simulink model "Brown_6DOF_Sim_Wrapper_EUL"  (R2025b)
settings: Solver=VariableStepAuto  StartTime=0.0  StopTime=10  RelTol=1e-3
values from neighbouring files (symbols this model uses):
  controller_airspeed_cmd_base = norm(V_init)    [Brown_6DOF_Init_main.m]    (also in Full_Sim_Init.m; Init_Main.m)
  controller_airspeed_step = 0.0    (= 0)    [Brown_6DOF_Init_main.m]    (also in Full_Sim_Init.m; Init_Main.m)
  controller_bank_cmd_base = eul_init(1)    [Brown_6DOF_Init_main.m]    (also in Full_Sim_Init.m; Init_Main.m)
  controller_bank_step = 0.0    (= 0)    [Brown_6DOF_Init_main.m]    (also in Full_Sim_Init.m; Init_Main.m)
  controller_enable = false    [Brown_6DOF_Init_main.m]    (also in Full_Sim_Init.m; Init_Main.m; Run_Main.m)
  controller_integrator_limit = 200.0    (= 200)    [Brown_6DOF_Init_main.m]    (also in Full_Sim_Init.m; Init_Main.m)
  controller_k_p_damp = 0.0    (= 0)    [Brown_6DOF_Init_main.m]    (also in Full_Sim_Init.m; Init_Main.m)
  controller_k_phi_i = 0.0    (= 0)    [Brown_6DOF_Init_main.m]    (also in Full_Sim_Init.m; Init_Main.m)
  controller_k_phi_p = 0.0    (= 0)    [Brown_6DOF_Init_main.m]    (also in Full_Sim_Init.m; Init_Main.m)
  controller_k_q_damp = 0.0    (= 0)    [Brown_6DOF_Init_main.m]    (also in Full_Sim_Init.m; Init_Main.m)
  controller_k_r_damp = 0.0    (= 0)    [Brown_6DOF_Init_main.m]    (also in Full_Sim_Init.m; Init_Main.m)
  controller_k_v_i = 0.0    (= 0)    [Brown_6DOF_Init_main.m]    (also in Full_Sim_Init.m; Init_Main.m)
  controller_k_v_p = 0.0    (= 0)    [Brown_6DOF_Init_main.m]    (also in Full_Sim_Init.m; Init_Main.m)
  controller_mode = 0    [Brown_6DOF_Init_main.m]    (also in Full_Sim_Init.m; Init_Main.m = 1; Run_Main.m = 1)
  controller_rpm_delta_limit = 2000.0    (= 2000)    [Brown_6DOF_Init_main.m]    (also in Full_Sim_Init.m; Init_Main.m)
  controller_sample_time = 0.01    [Brown_6DOF_Init_main.m]    (also in Full_Sim_Init.m; HW356_simple_demos_live_source.m; Init_Main.m)
  controller_step_time = 1.0    (= 1)    [Brown_6DOF_Init_main.m]    (also in Full_Sim_Init.m; Init_Main.m)
  controller_surface_limit_rad = deg2rad(25.0)    [Brown_6DOF_Init_main.m]    (also in Full_Sim_Init.m; Init_Main.m)
  controller_trim_delta_a = 0.0    (= 0)    [Brown_6DOF_Init_main.m]    (also in Full_Sim_Init.m; Init_Main.m)
  controller_trim_delta_e = 0.0    (= 0)    [Brown_6DOF_Init_main.m]    (also in Full_Sim_Init.m; Init_Main.m)
  controller_trim_delta_f = 0.0    (= 0)    [Brown_6DOF_Init_main.m]    (also in Full_Sim_Init.m; Init_Main.m)
  controller_trim_delta_r = 0.0    (= 0)    [Brown_6DOF_Init_main.m]    (also in Full_Sim_Init.m; Init_Main.m)
  controller_trim_motor_rpm_cmd = Motor_RPMs(:)    [Brown_6DOF_Init_main.m]    (also in Full_Sim_Init.m = zeros(12, 1); Init_Main.m = zeros(4, 1))
  controller_trim_tilt_angles_cmd = Tilt_angles(:)    [Brown_6DOF_Init_main.m]    (also in Full_Sim_Init.m = front_tilt_group * ones(6, 1); Init_Main.m = front_tilt_group * ones(numel(Tilt_angles), 1))
  estimator_enable = true    [Brown_6DOF_Init_main.m]    (also in Full_Sim_Init.m)
  estimator_init_eul = eul_init    [Brown_6DOF_Init_main.m]    (also in Full_Sim_Init.m)
  estimator_k_acc = 3.0    (= 3)    [Brown_6DOF_Init_main.m]    (also in Full_Sim_Init.m)
  estimator_k_att = 0.0    (= 0)    [Brown_6DOF_Init_main.m]    (also in Full_Sim_Init.m)
  estimator_k_mag = 1.5    [Brown_6DOF_Init_main.m]    (also in Full_Sim_Init.m)
  estimator_sample_time = controller_sample_time    (= 0.01)    [Brown_6DOF_Init_main.m]    (also in Full_Sim_Init.m)
  mag_ned = [0.23; 0.00; 0.43]    [Brown_6DOF_Init_main.m]    (also in Full_Sim_Init.m)
  sensor_accel_bias = zeros(3, 1)    [Brown_6DOF_Init_main.m]    (also in Full_Sim_Init.m; Init_Main.m = [0; 0; 0])
  sensor_accel_sigma = [0.05; 0.05; 0.05]    [Brown_6DOF_Init_main.m]    (also in Full_Sim_Init.m; Init_Main.m = [0; 0; 0])
  sensor_airdata_bias = zeros(3, 1)    [Brown_6DOF_Init_main.m]    (also in Full_Sim_Init.m; Init_Main.m = [0; 0; 0])
  sensor_airdata_sigma = [0.20; deg2rad(0.10); deg2rad(0.10)]    [Brown_6DOF_Init_main.m]    (also in Full_Sim_Init.m; Init_Main.m = [0; 0; 0])
  sensor_attitude_bias = zeros(3, 1)    [Brown_6DOF_Init_main.m]    (also in Full_Sim_Init.m)
  sensor_attitude_sigma = deg2rad([0.10; 0.10; 0.15])    [Brown_6DOF_Init_main.m]    (also in Full_Sim_Init.m)
  sensor_enable_bias = true    [Brown_6DOF_Init_main.m]    (also in Full_Sim_Init.m)
  sensor_enable_noise = true    [Brown_6DOF_Init_main.m]    (also in Full_Sim_Init.m)
  sensor_gps_pos_bias = zeros(3, 1)    [Brown_6DOF_Init_main.m]    (also in Full_Sim_Init.m)
  sensor_gps_pos_sigma = [0.50; 0.50; 0.50]    [Brown_6DOF_Init_main.m]    (also in Full_Sim_Init.m)
  sensor_gps_vel_bias = zeros(3, 1)    [Brown_6DOF_Init_main.m]    (also in Full_Sim_Init.m)
  sensor_gps_vel_sigma = [0.05; 0.05; 0.05]    [Brown_6DOF_Init_main.m]    (also in Full_Sim_Init.m)
  sensor_gyro_bias = zeros(3, 1)    [Brown_6DOF_Init_main.m]    (also in Full_Sim_Init.m; Init_Main.m = [0; 0; 0])
  sensor_gyro_sigma = deg2rad([0.05; 0.05; 0.05])    [Brown_6DOF_Init_main.m]    (also in Full_Sim_Init.m; Init_Main.m = [0; 0; 0])
  sensor_mag_bias = zeros(3, 1)    [Brown_6DOF_Init_main.m]    (also in Full_Sim_Init.m; Init_Main.m = [0; 0; 0])
  sensor_mag_sigma = [0.005; 0.005; 0.005]    [Brown_6DOF_Init_main.m]    (also in Full_Sim_Init.m; Init_Main.m = [0; 0; 0])
  sensor_sample_time = controller_sample_time    (= 0.01)    [Brown_6DOF_Init_main.m]    (also in Full_Sim_Init.m; Init_Main.m)
undefined symbols (not defined in the file or in its folder): trim_front_collective_rpm, trim_rear_collective_rpm
settings Model: Creator=zbrown  LastModifiedBy=zbrown

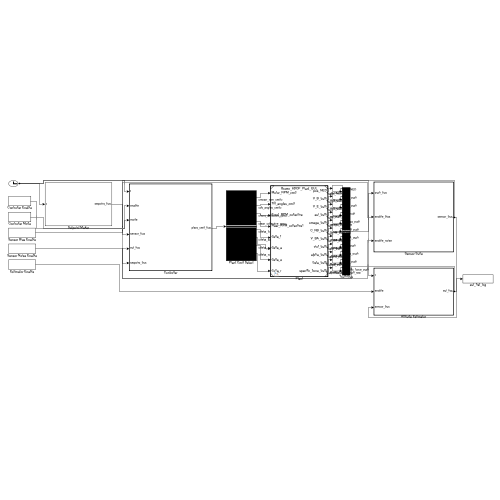
[thumbnail: Simulink's stored preview of the top-level diagram]
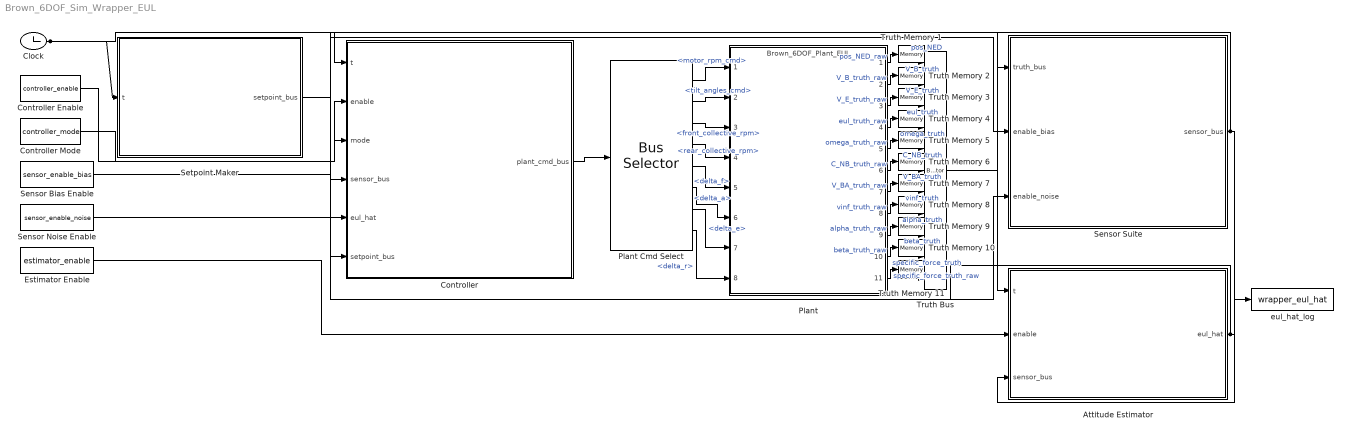
== system Brown_6DOF_Sim_Wrapper_EUL ==
  Attitude Estimator : Subsystem  TreatAsAtomicUnit=on  SystemSampleTime=estimator_sample_time
  Clock : Clock
  Controller : Subsystem  TreatAsAtomicUnit=on  SystemSampleTime=controller_sample_time
  Controller Enable : Constant  Value=controller_enable
  Controller Mode : Constant  Value=controller_mode
  Estimator Enable : Constant  Value=estimator_enable
  Plant : ModelReference  ModelNameDialog=Brown_6DOF_Plant_EUL  SimulationMode=Normal  ModelReferenceVersion=1.34
  Plant Cmd Select : BusSelector  OutputSignals=motor_rpm_cmd,tilt_angles_cmd,front_collective_rpm,rear_collective_rpm,delta_f,delta_a,delta_e,delta_r
  Sensor Bias Enable : Constant  Value=sensor_enable_bias
  Sensor Noise Enable : Constant  Value=sensor_enable_noise
  Sensor Suite : Subsystem  TreatAsAtomicUnit=on  SystemSampleTime=sensor_sample_time
  Setpoint Maker : Subsystem
  Truth Bus : BusCreator  Inputs=11
  Truth Memory {1..11} (11 alike) : Memory
  eul_hat_log : ToWorkspace  VariableName=wrapper_eul_hat  SampleTime=-1
  wires:
  Clock/1 -> Setpoint Maker/1(t), Controller/1(t), Attitude Estimator/1(t)
  Controller Enable/1 -> Controller/2(enable)
  Controller Mode/1 -> Controller/3(mode)
  Setpoint Maker/1(setpoint_bus) -> Controller/6(setpoint_bus)
  Controller/1(plant_cmd_bus) -> Plant Cmd Select/1
  Plant Cmd Select/1 -> Plant/1  "<motor_rpm_cmd>"
  Plant Cmd Select/2 -> Plant/2  "<tilt_angles_cmd>"
  Plant Cmd Select/3 -> Plant/3  "<front_collective_rpm>"
  Plant Cmd Select/4 -> Plant/4  "<rear_collective_rpm>"
  Plant Cmd Select/5 -> Plant/5  "<delta_f>"
  Plant Cmd Select/6 -> Plant/6  "<delta_a>"
  Plant Cmd Select/7 -> Plant/7  "<delta_e>"
  Plant Cmd Select/8 -> Plant/8  "<delta_r>"
  Plant/1 -> Truth Memory 1/1  "pos_NED_raw"
  Truth Memory 1/1 -> Truth Bus/1  "pos_NED"
  Plant/2 -> Truth Memory 2/1  "V_B_truth_raw"
  Truth Memory 2/1 -> Truth Bus/2  "V_B_truth"
  Plant/3 -> Truth Memory 3/1  "V_E_truth_raw"
  Truth Memory 3/1 -> Truth Bus/3  "V_E_truth"
  Plant/4 -> Truth Memory 4/1  "eul_truth_raw"
  Truth Memory 4/1 -> Truth Bus/4  "eul_truth"
  Plant/5 -> Truth Memory 5/1  "omega_truth_raw"
  Truth Memory 5/1 -> Truth Bus/5  "omega_truth"
  Plant/6 -> Truth Memory 6/1  "C_NB_truth_raw"
  Truth Memory 6/1 -> Truth Bus/6  "C_NB_truth"
  Plant/7 -> Truth Memory 7/1  "V_BA_truth_raw"
  Truth Memory 7/1 -> Truth Bus/7  "V_BA_truth"
  Plant/8 -> Truth Memory 8/1  "vinf_truth_raw"
  Truth Memory 8/1 -> Truth Bus/8  "vinf_truth"
  Plant/9 -> Truth Memory 9/1  "alpha_truth_raw"
  Truth Memory 9/1 -> Truth Bus/9  "alpha_truth"
  Plant/10 -> Truth Memory 10/1  "beta_truth_raw"
  Truth Memory 10/1 -> Truth Bus/10  "beta_truth"
  Plant/11 -> Truth Memory 11/1  "specific_force_truth_raw"
  Truth Memory 11/1 -> Truth Bus/11  "specific_force_truth"
  Truth Bus/1 -> Sensor Suite/1(truth_bus)
  Sensor Bias Enable/1 -> Sensor Suite/2(enable_bias)
  Sensor Noise Enable/1 -> Sensor Suite/3(enable_noise)
  Sensor Suite/1(sensor_bus) -> Attitude Estimator/3(sensor_bus), Controller/4(sensor_bus)
  Estimator Enable/1 -> Attitude Estimator/2(enable)
  Attitude Estimator/1(eul_hat) -> Controller/5(eul_hat), eul_hat_log/1

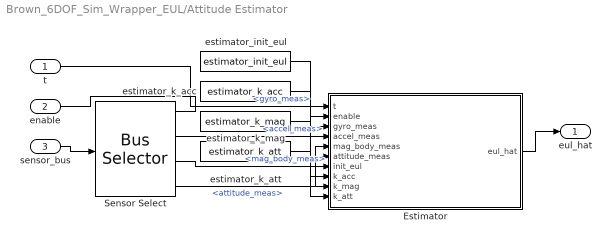
== system Brown_6DOF_Sim_Wrapper_EUL/Attitude Estimator ==
  t : Inport
  enable : Inport  Port=2
  sensor_bus : Inport  Port=3
  Estimator : MATLAB Function  TreatAsAtomicUnit=on
  Sensor Select : BusSelector  OutputSignals=gyro_meas,accel_meas,mag_body_meas,attitude_meas
  estimator_init_eul : Constant  Value=estimator_init_eul
  estimator_k_acc : Constant  Value=estimator_k_acc
  estimator_k_att : Constant  Value=estimator_k_att
  estimator_k_mag : Constant  Value=estimator_k_mag
  eul_hat : Outport
  wires:
  ? -> ?
  t/1 -> Estimator/1(t)
  enable/1 -> Estimator/2(enable)
  sensor_bus/1 -> Sensor Select/1
  Sensor Select/1 -> Estimator/3(gyro_meas)  "<gyro_meas>"
  Sensor Select/2 -> Estimator/4(accel_meas)  "<accel_meas>"
  Sensor Select/3 -> Estimator/5(mag_body_meas)  "<mag_body_meas>"
  Sensor Select/4 -> Estimator/6(attitude_meas)  "<attitude_meas>"
  estimator_init_eul/1 -> Estimator/7(init_eul)
  estimator_k_acc/1 -> Estimator/8(k_acc)
  estimator_k_mag/1 -> Estimator/9(k_mag)
  estimator_k_att/1 -> Estimator/10(k_att)
  Estimator/1(eul_hat) -> eul_hat/1

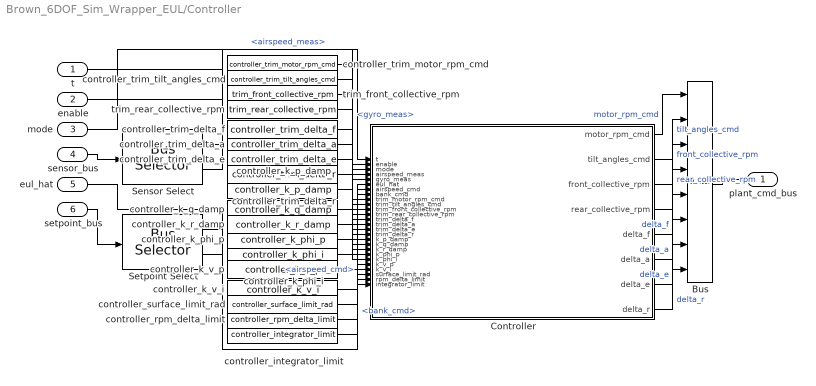
== system Brown_6DOF_Sim_Wrapper_EUL/Controller ==
  t : Inport
  enable : Inport  Port=2
  mode : Inport  Port=3
  sensor_bus : Inport  Port=4
  eul_hat : Inport  Port=5
  setpoint_bus : Inport  Port=6
  Bus : BusCreator  Inputs=8
  Controller : MATLAB Function  TreatAsAtomicUnit=on
  Sensor Select : BusSelector  OutputSignals=airspeed_meas,gyro_meas
  Setpoint Select : BusSelector  OutputSignals=airspeed_cmd,bank_cmd
  controller_integrator_limit : Constant  Value=controller_integrator_limit
  controller_k_p_damp : Constant  Value=controller_k_p_damp
  controller_k_phi_i : Constant  Value=controller_k_phi_i
  controller_k_phi_p : Constant  Value=controller_k_phi_p
  controller_k_q_damp : Constant  Value=controller_k_q_damp
  controller_k_r_damp : Constant  Value=controller_k_r_damp
  controller_k_v_i : Constant  Value=controller_k_v_i
  controller_k_v_p : Constant  Value=controller_k_v_p
  controller_rpm_delta_limit : Constant  Value=controller_rpm_delta_limit
  controller_surface_limit_rad : Constant  Value=controller_surface_limit_rad
  controller_trim_delta_a : Constant  Value=controller_trim_delta_a
  controller_trim_delta_e : Constant  Value=controller_trim_delta_e
  controller_trim_delta_f : Constant  Value=controller_trim_delta_f
  controller_trim_delta_r : Constant  Value=controller_trim_delta_r
  controller_trim_motor_rpm_cmd : Constant  Value=controller_trim_motor_rpm_cmd
  controller_trim_tilt_angles_cmd : Constant  Value=controller_trim_tilt_angles_cmd
  trim_front_collective_rpm : Constant  Value=trim_front_collective_rpm
  trim_rear_collective_rpm : Constant  Value=trim_rear_collective_rpm
  plant_cmd_bus : Outport
  wires:
  ? -> ?
  t/1 -> Controller/1(t)
  enable/1 -> Controller/2(enable)
  mode/1 -> Controller/3(mode)
  sensor_bus/1 -> Sensor Select/1
  setpoint_bus/1 -> Setpoint Select/1
  eul_hat/1 -> Controller/6(eul_hat)
  Sensor Select/1 -> Controller/4(airspeed_meas)  "<airspeed_meas>"
  Sensor Select/2 -> Controller/5(gyro_meas)  "<gyro_meas>"
  Setpoint Select/1 -> Controller/7(airspeed_cmd)  "<airspeed_cmd>"
  Setpoint Select/2 -> Controller/8(bank_cmd)  "<bank_cmd>"
  controller_trim_motor_rpm_cmd/1 -> Controller/9(trim_motor_rpm_cmd)
  controller_trim_tilt_angles_cmd/1 -> Controller/10(trim_tilt_angles_cmd)
  trim_front_collective_rpm/1 -> Controller/11(trim_front_collective_rpm)
  trim_rear_collective_rpm/1 -> Controller/12(trim_rear_collective_rpm)
  controller_trim_delta_f/1 -> Controller/13(trim_delta_f)
  controller_trim_delta_a/1 -> Controller/14(trim_delta_a)
  controller_trim_delta_e/1 -> Controller/15(trim_delta_e)
  controller_trim_delta_r/1 -> Controller/16(trim_delta_r)
  controller_k_p_damp/1 -> Controller/17(k_p_damp)
  controller_k_q_damp/1 -> Controller/18(k_q_damp)
  controller_k_r_damp/1 -> Controller/19(k_r_damp)
  controller_k_phi_p/1 -> Controller/20(k_phi_p)
  controller_k_phi_i/1 -> Controller/21(k_phi_i)
  controller_k_v_p/1 -> Controller/22(k_v_p)
  controller_k_v_i/1 -> Controller/23(k_v_i)
  controller_surface_limit_rad/1 -> Controller/24(surface_limit_rad)
  controller_rpm_delta_limit/1 -> Controller/25(rpm_delta_limit)
  controller_integrator_limit/1 -> Controller/26(integrator_limit)
  Controller/1(motor_rpm_cmd) -> Bus/1  "motor_rpm_cmd"
  Controller/2(tilt_angles_cmd) -> Bus/2  "tilt_angles_cmd"
  Controller/3(front_collective_rpm) -> Bus/3  "front_collective_rpm"
  Controller/4(rear_collective_rpm) -> Bus/4  "rear_collective_rpm"
  Controller/5(delta_f) -> Bus/5  "delta_f"
  Controller/6(delta_a) -> Bus/6  "delta_a"
  Controller/7(delta_e) -> Bus/7  "delta_e"
  Controller/8(delta_r) -> Bus/8  "delta_r"
  Bus/1 -> plant_cmd_bus/1

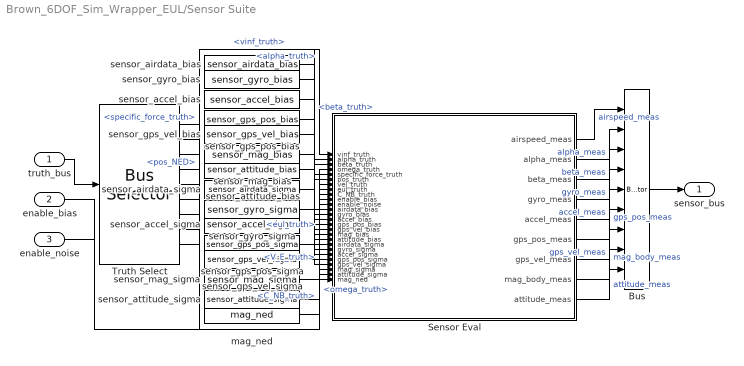
== system Brown_6DOF_Sim_Wrapper_EUL/Sensor Suite ==
  truth_bus : Inport
  enable_bias : Inport  Port=2
  enable_noise : Inport  Port=3
  Bus : BusCreator  Inputs=9
  Sensor Eval : MATLAB Function  TreatAsAtomicUnit=on
  Truth Select : BusSelector  OutputSignals=vinf_truth,alpha_truth,beta_truth,omega_truth,specific_force_truth,pos_NED,V_E_truth,eul_truth,C_NB_truth
  mag_ned : Constant  Value=mag_ned
  sensor_accel_bias : Constant  Value=sensor_accel_bias
  sensor_accel_sigma : Constant  Value=sensor_accel_sigma
  sensor_airdata_bias : Constant  Value=sensor_airdata_bias
  sensor_airdata_sigma : Constant  Value=sensor_airdata_sigma
  sensor_attitude_bias : Constant  Value=sensor_attitude_bias
  sensor_attitude_sigma : Constant  Value=sensor_attitude_sigma
  sensor_gps_pos_bias : Constant  Value=sensor_gps_pos_bias
  sensor_gps_pos_sigma : Constant  Value=sensor_gps_pos_sigma
  sensor_gps_vel_bias : Constant  Value=sensor_gps_vel_bias
  sensor_gps_vel_sigma : Constant  Value=sensor_gps_vel_sigma
  sensor_gyro_bias : Constant  Value=sensor_gyro_bias
  sensor_gyro_sigma : Constant  Value=sensor_gyro_sigma
  sensor_mag_bias : Constant  Value=sensor_mag_bias
  sensor_mag_sigma : Constant  Value=sensor_mag_sigma
  sensor_bus : Outport
  wires:
  ? -> ?
  truth_bus/1 -> Truth Select/1
  Truth Select/1 -> Sensor Eval/1(vinf_truth)  "<vinf_truth>"
  Truth Select/2 -> Sensor Eval/2(alpha_truth)  "<alpha_truth>"
  Truth Select/3 -> Sensor Eval/3(beta_truth)  "<beta_truth>"
  Truth Select/4 -> Sensor Eval/4(omega_truth)  "<omega_truth>"
  Truth Select/5 -> Sensor Eval/5(specific_force_truth)  "<specific_force_truth>"
  Truth Select/6 -> Sensor Eval/6(pos_truth)  "<pos_NED>"
  Truth Select/7 -> Sensor Eval/7(vel_truth)  "<V_E_truth>"
  Truth Select/8 -> Sensor Eval/8(eul_truth)  "<eul_truth>"
  Truth Select/9 -> Sensor Eval/9(C_NB_truth)  "<C_NB_truth>"
  enable_bias/1 -> Sensor Eval/10(enable_bias)
  enable_noise/1 -> Sensor Eval/11(enable_noise)
  sensor_airdata_bias/1 -> Sensor Eval/12(airdata_bias)
  sensor_gyro_bias/1 -> Sensor Eval/13(gyro_bias)
  sensor_accel_bias/1 -> Sensor Eval/14(accel_bias)
  sensor_gps_pos_bias/1 -> Sensor Eval/15(gps_pos_bias)
  sensor_gps_vel_bias/1 -> Sensor Eval/16(gps_vel_bias)
  sensor_mag_bias/1 -> Sensor Eval/17(mag_bias)
  sensor_attitude_bias/1 -> Sensor Eval/18(attitude_bias)
  sensor_airdata_sigma/1 -> Sensor Eval/19(airdata_sigma)
  sensor_gyro_sigma/1 -> Sensor Eval/20(gyro_sigma)
  sensor_accel_sigma/1 -> Sensor Eval/21(accel_sigma)
  sensor_gps_pos_sigma/1 -> Sensor Eval/22(gps_pos_sigma)
  sensor_gps_vel_sigma/1 -> Sensor Eval/23(gps_vel_sigma)
  sensor_mag_sigma/1 -> Sensor Eval/24(mag_sigma)
  sensor_attitude_sigma/1 -> Sensor Eval/25(attitude_sigma)
  mag_ned/1 -> Sensor Eval/26(mag_ned)
  Sensor Eval/1(airspeed_meas) -> Bus/1  "airspeed_meas"
  Sensor Eval/2(alpha_meas) -> Bus/2  "alpha_meas"
  Sensor Eval/3(beta_meas) -> Bus/3  "beta_meas"
  Sensor Eval/4(gyro_meas) -> Bus/4  "gyro_meas"
  Sensor Eval/5(accel_meas) -> Bus/5  "accel_meas"
  Sensor Eval/6(gps_pos_meas) -> Bus/6  "gps_pos_meas"
  Sensor Eval/7(gps_vel_meas) -> Bus/7  "gps_vel_meas"
  Sensor Eval/8(mag_body_meas) -> Bus/8  "mag_body_meas"
  Sensor Eval/9(attitude_meas) -> Bus/9  "attitude_meas"
  Bus/1 -> sensor_bus/1

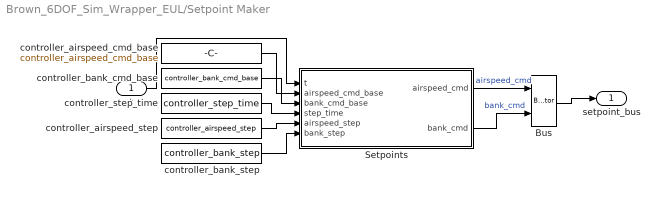
== system Brown_6DOF_Sim_Wrapper_EUL/Setpoint Maker ==
  t : Inport
  Bus : BusCreator  Inputs=2
  Setpoints : MATLAB Function  TreatAsAtomicUnit=on
  controller_airspeed_cmd_base : Constant  Value=controller_airspeed_cmd_base
  controller_airspeed_step : Constant  Value=controller_airspeed_step
  controller_bank_cmd_base : Constant  Value=controller_bank_cmd_base
  controller_bank_step : Constant  Value=controller_bank_step
  controller_step_time : Constant  Value=controller_step_time
  setpoint_bus : Outport
  wires:
  ? -> ?
  t/1 -> Setpoints/1(t)
  controller_airspeed_cmd_base/1 -> Setpoints/2(airspeed_cmd_base)
  controller_bank_cmd_base/1 -> Setpoints/3(bank_cmd_base)
  controller_step_time/1 -> Setpoints/4(step_time)
  controller_airspeed_step/1 -> Setpoints/5(airspeed_step)
  controller_bank_step/1 -> Setpoints/6(bank_step)
  Setpoints/1(airspeed_cmd) -> Bus/1  "airspeed_cmd"
  Setpoints/2(bank_cmd) -> Bus/2  "bank_cmd"
  Bus/1 -> setpoint_bus/1

== matlab function Brown_6DOF_Sim_Wrapper_EUL/Attitude Estimator/Estimator ==
  data: t input; eul_hat output; enable input; gyro_meas input; accel_meas input; mag_body_meas input; attitude_meas input; init_eul input; k_acc input; k_mag input; k_att input
function eul_hat = fcn(t, enable, gyro_meas, accel_meas, mag_body_meas, attitude_meas, init_eul, k_acc, k_mag, k_att)
%#codegen
eul_hat = attitude_complementary_step(t, enable, gyro_meas, accel_meas, mag_body_meas, attitude_meas, init_eul, k_acc, k_mag, k_att);
end

== matlab function Brown_6DOF_Sim_Wrapper_EUL/Controller/Controller ==
  data: t input; motor_rpm_cmd output; enable input; mode input; airspeed_meas input; gyro_meas input; eul_hat input; airspeed_cmd input; bank_cmd input; trim_motor_rpm_cmd input; trim_tilt_angles_cmd input; trim_front_collective_rpm input; trim_rear_collective_rpm input; trim_delta_f input; trim_delta_a input; trim_delta_e input; trim_delta_r input; k_p_damp input; k_q_damp input; k_r_damp input; k_phi_p input; k_phi_i input; k_v_p input; k_v_i input; surface_limit_rad input; rpm_delta_limit input; integrator_limit input; tilt_angles_cmd output; front_collective_rpm output; rear_collective_rpm output; delta_f output; delta_a output; delta_e output; delta_r output
function [motor_rpm_cmd, tilt_angles_cmd, front_collective_rpm, rear_collective_rpm, delta_f, delta_a, delta_e, delta_r] = fcn(t, enable, mode, airspeed_meas, gyro_meas, eul_hat, airspeed_cmd, bank_cmd, trim_motor_rpm_cmd, trim_tilt_angles_cmd, trim_front_collective_rpm, trim_rear_collective_rpm, trim_delta_f, trim_delta_a, trim_delta_e, trim_delta_r, k_p_damp, k_q_damp, k_r_damp, k_phi_p, k_phi_i, k_v_p, k_v_i, surface_limit_rad, rpm_delta_limit, integrator_limit)
%#codegen
[motor_rpm_cmd, tilt_angles_cmd, front_collective_rpm, rear_collective_rpm, delta_f, delta_a, delta_e, delta_r] = wrapper_controller_actual_cmd_step(t, enable, mode, airspeed_meas, gyro_meas, eul_hat, airspeed_cmd, bank_cmd, trim_motor_rpm_cmd, trim_tilt_angles_cmd, trim_front_collective_rpm, trim_rear_collective_rpm, trim_delta_f, trim_delta_a, trim_delta_e, trim_delta_r, k_p_damp, k_q_damp, k_r_damp, k_phi_p, k_phi_i, k_v_p, k_v_i, surface_limit_rad, rpm_delta_limit, integrator_limit);
end

== matlab function Brown_6DOF_Sim_Wrapper_EUL/Setpoint Maker/Setpoints ==
  data: t input; airspeed_cmd output; airspeed_cmd_base input; bank_cmd_base input; step_time input; airspeed_step input; bank_step input; bank_cmd output
function [airspeed_cmd, bank_cmd] = fcn(t, airspeed_cmd_base, bank_cmd_base, step_time, airspeed_step, bank_step)
%#codegen
[airspeed_cmd, bank_cmd] = setpoint_schedule_step(t, airspeed_cmd_base, bank_cmd_base, step_time, airspeed_step, bank_step);
end

== matlab function Brown_6DOF_Sim_Wrapper_EUL/Sensor Suite/Sensor Eval ==
  data: vinf_truth input; airspeed_meas output; alpha_truth input; beta_truth input; omega_truth input; specific_force_truth input; pos_truth input; vel_truth input; eul_truth input; C_NB_truth input; enable_bias input; enable_noise input; airdata_bias input; gyro_bias input; accel_bias input; gps_pos_bias input; gps_vel_bias input; mag_bias input; attitude_bias input; airdata_sigma input; gyro_sigma input; accel_sigma input; gps_pos_sigma input; gps_vel_sigma input; mag_sigma input; attitude_sigma input; mag_ned input; alpha_meas output; beta_meas output; gyro_meas output; accel_meas output; gps_pos_meas output; gps_vel_meas output; mag_body_meas output; attitude_meas output
function [airspeed_meas, alpha_meas, beta_meas, gyro_meas, accel_meas, gps_pos_meas, gps_vel_meas, mag_body_meas, attitude_meas] = fcn(vinf_truth, alpha_truth, beta_truth, omega_truth, specific_force_truth, pos_truth, vel_truth, eul_truth, C_NB_truth, enable_bias, enable_noise, airdata_bias, gyro_bias, accel_bias, gps_pos_bias, gps_vel_bias, mag_bias, attitude_bias, airdata_sigma, gyro_sigma, accel_sigma, gps_pos_sigma, gps_vel_sigma, mag_sigma, attitude_sigma, mag_ned)
%#codegen
[airspeed_meas, alpha_meas, beta_meas, gyro_meas, accel_meas, gps_pos_meas, gps_vel_meas, mag_body_meas, attitude_meas] = sensor_suite_eval(vinf_truth, alpha_truth, beta_truth, omega_truth, specific_force_truth, pos_truth, vel_truth, eul_truth, C_NB_truth, enable_bias, enable_noise, airdata_bias, gyro_bias, accel_bias, gps_pos_bias, gps_vel_bias, mag_bias, attitude_bias, airdata_sigma, gyro_sigma, accel_sigma, gps_pos_sigma, gps_vel_sigma, mag_sigma, attitude_sigma, mag_ned);
end
